simulink model "lab3_p8"  (R2020a)
settings: Solver=VariableStepAuto  StartTime=0.0  StopTime=stop_time  RelTol=1e-3
InitFcn:
  | sm_callback_init.m
StopFcn:
  | sm_callback_stop
values from neighbouring files (symbols this model uses):
  mp = sm_init_control_signals(mp)    [sm_callback_init.m]
libraries: simulink x2
settings Model: Creator=Owner  LastModifiedBy=Owner
settings DataIOCC: ReturnWorkspaceOutputs=off

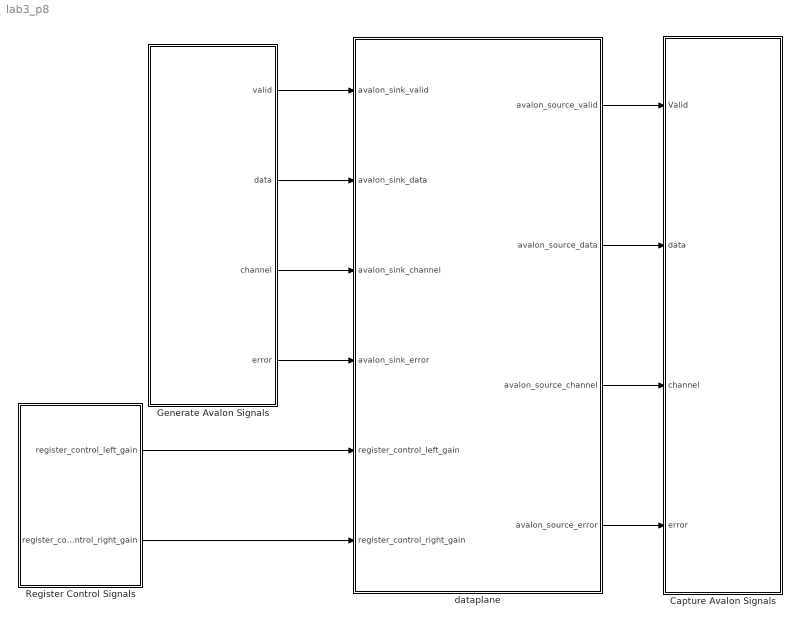
== system lab3_p8 ==
  Capture Avalon Signals : Subsystem
  Generate Avalon Signals : Subsystem
  Register Control Signals : Subsystem
  dataplane : Subsystem
  wires:
  Generate Avalon Signals/1(valid) -> dataplane/1(avalon_sink_valid)
  Generate Avalon Signals/2(data) -> dataplane/2(avalon_sink_data)
  Generate Avalon Signals/3(channel) -> dataplane/3(avalon_sink_channel)
  Generate Avalon Signals/4(error) -> dataplane/4(avalon_sink_error)
  dataplane/1(avalon_source_valid) -> Capture Avalon Signals/1(Valid)
  dataplane/2(avalon_source_data) -> Capture Avalon Signals/2(data)
  dataplane/3(avalon_source_channel) -> Capture Avalon Signals/3(channel)
  dataplane/4(avalon_source_error) -> Capture Avalon Signals/4(error)
  Register Control Signals/2(register_control_right_gain) -> dataplane/6(register_control_right_gain)
  Register Control Signals/1(register_control_left_gain) -> dataplane/5(register_control_left_gain)

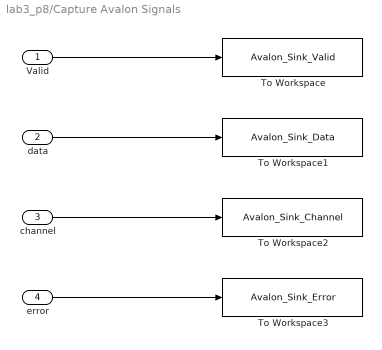
== system lab3_p8/Capture Avalon Signals ==
  Valid : Inport
  data : Inport  Port=2
  channel : Inport  Port=3
  error : Inport  Port=4
  To Workspace : ToWorkspace  VariableName=Avalon_Sink_Valid  SampleTime=-1
      settings: Save2DSignal=2-D array (concatenate along first dimension)
  To Workspace1 : ToWorkspace  VariableName=Avalon_Sink_Data  SampleTime=-1
      settings: Save2DSignal=2-D array (concatenate along first dimension)
  To Workspace2 : ToWorkspace  VariableName=Avalon_Sink_Channel  SampleTime=-1
      settings: Save2DSignal=2-D array (concatenate along first dimension)
  To Workspace3 : ToWorkspace  VariableName=Avalon_Sink_Error  SampleTime=-1
      settings: Save2DSignal=2-D array (concatenate along first dimension)
  wires:
  Valid/1 -> To Workspace/1
  data/1 -> To Workspace1/1
  channel/1 -> To Workspace2/1
  error/1 -> To Workspace3/1

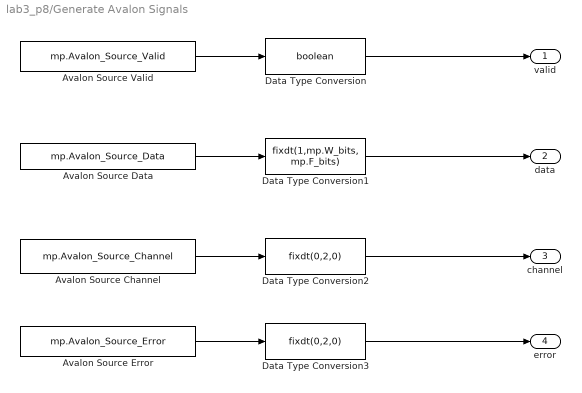
== system lab3_p8/Generate Avalon Signals ==
  Avalon Source Channel : FromWorkspace  VariableName=mp.Avalon_Source_Channel  OutDataTypeStr=double  SampleTime=mp.Ts_system
  Avalon Source Data : FromWorkspace  VariableName=mp.Avalon_Source_Data  OutDataTypeStr=double  SampleTime=mp.Ts_system
  Avalon Source Error : FromWorkspace  VariableName=mp.Avalon_Source_Error  OutDataTypeStr=double  SampleTime=mp.Ts_system
  Avalon Source Valid : FromWorkspace  VariableName=mp.Avalon_Source_Valid  OutDataTypeStr=double  SampleTime=mp.Ts_system
  Data Type Conversion : DataTypeConversion  OutDataTypeStr=boolean  RndMeth=Nearest
  Data Type Conversion1 : DataTypeConversion  OutDataTypeStr=fixdt(1,mp.W_bits, mp.F_bits)  RndMeth=Nearest
  Data Type Conversion2 : DataTypeConversion  OutDataTypeStr=fixdt(0,2,0)  RndMeth=Nearest
  Data Type Conversion3 : DataTypeConversion  OutDataTypeStr=fixdt(0,2,0)  RndMeth=Nearest
  valid : Outport
  data : Outport  Port=2
  channel : Outport  Port=3
  error : Outport  Port=4
  wires:
  Data Type Conversion/1 -> valid/1
  Avalon Source Valid/1 -> Data Type Conversion/1
  Avalon Source Data/1 -> Data Type Conversion1/1
  Data Type Conversion1/1 -> data/1
  Data Type Conversion2/1 -> channel/1
  Avalon Source Channel/1 -> Data Type Conversion2/1
  Data Type Conversion3/1 -> error/1
  Avalon Source Error/1 -> Data Type Conversion3/1

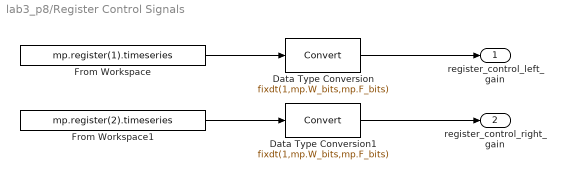
== system lab3_p8/Register Control Signals ==
  Data Type Conversion : DataTypeConversion  OutDataTypeStr=fixdt(1,mp.W_bits,mp.F_bits)
  Data Type Conversion1 : DataTypeConversion  OutDataTypeStr=fixdt(1,mp.W_bits,mp.F_bits)
  From Workspace : FromWorkspace  VariableName=mp.register(1).timeseries  OutDataTypeStr=double  SampleTime=mp.Ts_system
  From Workspace1 : FromWorkspace  VariableName=mp.register(2).timeseries  OutDataTypeStr=double  SampleTime=mp.Ts_system
  register_control_left_gain : Outport
  register_control_right_gain : Outport  Port=2
  wires:
  From Workspace/1 -> Data Type Conversion/1
  Data Type Conversion/1 -> register_control_left_gain/1
  From Workspace1/1 -> Data Type Conversion1/1
  Data Type Conversion1/1 -> register_control_right_gain/1

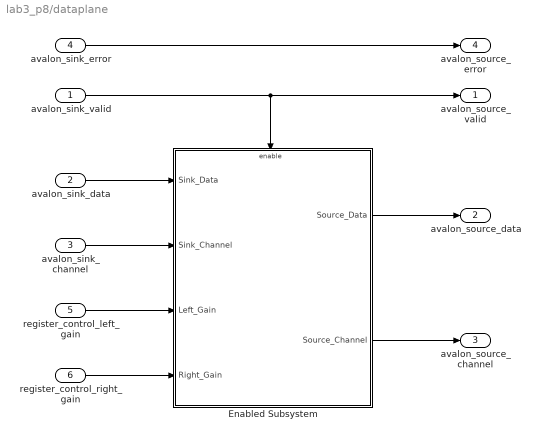
== system lab3_p8/dataplane ==
  avalon_sink_valid : Inport
  avalon_sink_data : Inport  Port=2
  avalon_sink_channel : Inport  Port=3
  avalon_sink_error : Inport  Port=4
  register_control_left_gain : Inport  Port=5
  register_control_right_gain : Inport  Port=6
  Enabled Subsystem : Subsystem  TreatAsAtomicUnit=on
  avalon_source_valid : Outport  VectorParamsAs1DForOutWhenUnconnected=off
  avalon_source_data : Outport  Port=2  VectorParamsAs1DForOutWhenUnconnected=off
  avalon_source_channel : Outport  Port=3  VectorParamsAs1DForOutWhenUnconnected=off
  avalon_source_error : Outport  Port=4  VectorParamsAs1DForOutWhenUnconnected=off
  wires:
  avalon_sink_error/1 -> avalon_source_error/1
  avalon_sink_valid/1 -> avalon_source_valid/1, Enabled Subsystem/Enable
  Enabled Subsystem/1(Source_Data) -> avalon_source_data/1
  Enabled Subsystem/2(Source_Channel) -> avalon_source_channel/1
  avalon_sink_data/1 -> Enabled Subsystem/1(Sink_Data)
  avalon_sink_channel/1 -> Enabled Subsystem/2(Sink_Channel)
  register_control_right_gain/1 -> Enabled Subsystem/4(Right_Gain)
  register_control_left_gain/1 -> Enabled Subsystem/3(Left_Gain)

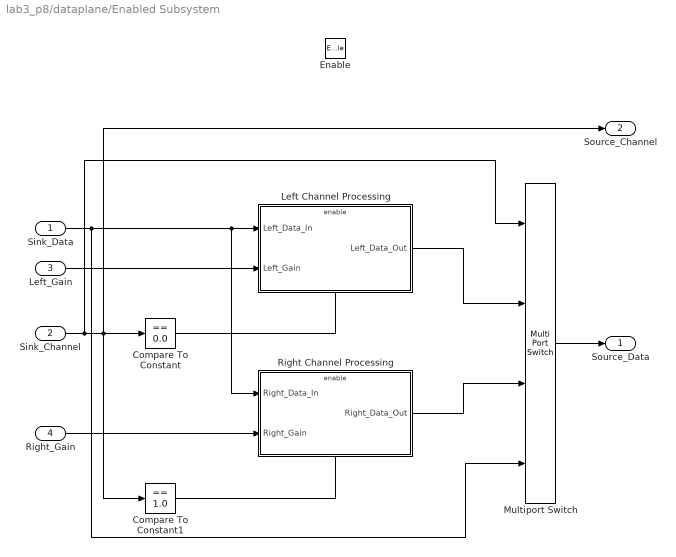
== system lab3_p8/dataplane/Enabled Subsystem ==
  Sink_Data : Inport
  Sink_Channel : Inport  Port=2
  Left_Gain : Inport  Port=3
  Right_Gain : Inport  Port=4
  Enable : EnablePort
  Compare To Constant : simulink/Logic and Bit Operations/Compare To Constant  relop===  const=0.0  OutDataTypeStr=boolean
  Compare To Constant1 : simulink/Logic and Bit Operations/Compare To Constant  relop===  const=1.0  OutDataTypeStr=boolean
  Left Channel Processing : Subsystem  TreatAsAtomicUnit=on
  Multiport Switch : MultiPortSwitch  DataPortOrder=Zero-based contiguous  zeroidx=on
  Right Channel Processing : Subsystem  TreatAsAtomicUnit=on
  Source_Data : Outport
  Source_Channel : Outport  Port=2
  wires:
  Sink_Data/1 -> Multiport Switch/4, Right Channel Processing/1(Right_Data_In), Left Channel Processing/1(Left_Data_In)
  Sink_Channel/1 -> Multiport Switch/1, Compare To Constant1/1, Source_Channel/1, Compare To Constant/1
  Left_Gain/1 -> Left Channel Processing/2(Left_Gain)
  Right_Gain/1 -> Right Channel Processing/2(Right_Gain)
  Compare To Constant1/1 -> Right Channel Processing/Enable
  Compare To Constant/1 -> Left Channel Processing/Enable
  Multiport Switch/1 -> Source_Data/1
  Left Channel Processing/1(Left_Data_Out) -> Multiport Switch/2
  Right Channel Processing/1(Right_Data_Out) -> Multiport Switch/3

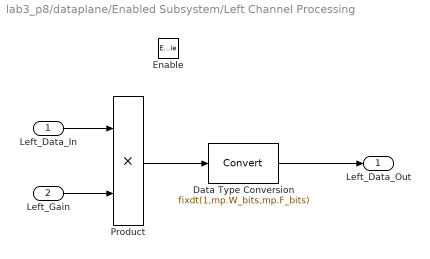
== system lab3_p8/dataplane/Enabled Subsystem/Left Channel Processing ==
  Left_Data_In : Inport
  Left_Gain : Inport  Port=2
  Enable : EnablePort
  Data Type Conversion : DataTypeConversion  OutDataTypeStr=fixdt(1,mp.W_bits,mp.F_bits)  RndMeth=Nearest
  Product : Product
  Left_Data_Out : Outport  InitialOutput=0  VectorParamsAs1DForOutWhenUnconnected=off
  wires:
  Left_Data_In/1 -> Product/1
  Left_Gain/1 -> Product/2
  Product/1 -> Data Type Conversion/1
  Data Type Conversion/1 -> Left_Data_Out/1

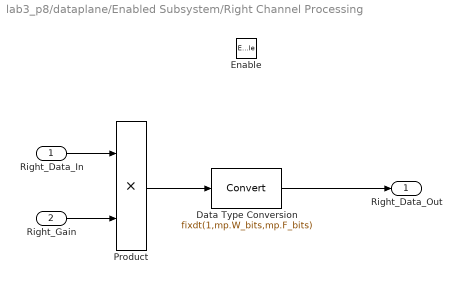
== system lab3_p8/dataplane/Enabled Subsystem/Right Channel Processing ==
  Right_Data_In : Inport
  Right_Gain : Inport  Port=2
  Enable : EnablePort
  Data Type Conversion : DataTypeConversion  OutDataTypeStr=fixdt(1,mp.W_bits,mp.F_bits)  RndMeth=Nearest
  Product : Product
  Right_Data_Out : Outport  InitialOutput=0  VectorParamsAs1DForOutWhenUnconnected=off
  wires:
  Product/1 -> Data Type Conversion/1
  Right_Data_In/1 -> Product/1
  Right_Gain/1 -> Product/2
  Data Type Conversion/1 -> Right_Data_Out/1
